simulink model "rtwdemo_sffor"  (Simulink 6.0)
settings: Solver=FixedStepDiscrete  StartTime=0.0  StopTime=10  FixedStep=1  RelTol=1e-3
PostLoadFcn:
  | rtwdemo_sffor_data
undefined symbols (not defined in the file or in its folder): P1, P2
libraries: rtwdemowidgets x2
settings Model: Creator=The MathWorks Inc.  LastModifiedBy=batserve  ExtModeAutoUpdateStatusClock=off  ProdHWDeviceType=32-bit Embedded Processor
settings DataIOCC: SaveOutput=off  SaveTime=off  SignalLoggingName=logsOut
settings OptimizationCC: InlineParams=on  EnforceIntegerDowncast=off  StateBitsets=on  DataBitsets=on  UseTempVars=on
settings DebuggingCC: CheckExecutionContextPreStartOutputMsg=on  CheckExecutionContextRuntimeOutputMsg=on  SolverPrmCheckMsg=none
settings HardwareCC: ProdHWDeviceType=32-bit Embedded Processor  TargetHWDeviceType=32-bit Generic  ProdEqTarget=off
settings ModelReferenceCC: UpdateModelReferenceTargets=IfOutOfDate
settings RTWCC: TLCOptions=-p0 -aWarnNonSaturatedBlocks=0  GenCodeOnly=on  Description=RTW Embedded Coder (auto configures for optimized floating-point code)  GenerateReport=on  RTWVerbose=off  ProcessScript=grt_make_rtw_hook  LaunchReport=on
settings CodeAppCC: ForceParamTrailComments=on
settings GRTTargetCC: MatFileLogging=off

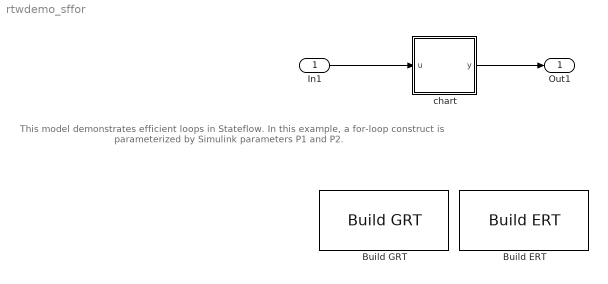
== system rtwdemo_sffor ==
  note: This model demonstrates efficient loops in Stateflow.  In this example,
      | a for-loop construct is parameterized by Simulink parameters P1 and P2.
  In1 : Inport  Port=1  DataType=single  LatchInput=off
  Build ERT : rtwdemowidgets/Build ERT  attrib_overrides={}
  Build GRT : rtwdemowidgets/Build GRT  attrib_overrides={}
  chart : Stateflow chart  PropExecContextAcrossSSBoundary=on
  Out1 : Outport
  wires:
  chart/1(y) -> Out1/1
  In1/1 -> chart/1(u)

== stateflow chart chart ==
  state f [function]
    (default) -> (junction 4) : {y=0;i=P1;}
    (junction 4) -> (junction 4) : [i<P2]{x=x+x*i;i++}
    (junction 4) -> (junction 5) : {y=u*x;}
  (default) -> (junction 6) : {f();}
  data: x temporary type(u) size=1; i local int8 size=1; P1 parameter inherited size=1; P2 parameter inherited size=1; y output type(u) size=1; u input inherited
